simulink model "Section2_b"  (R2023b)
settings: Solver=VariableStepAuto  StartTime=0.0  StopTime=20.0  RelTol=1e-3
settings Model: Creator=paria  LastModifiedBy=paria

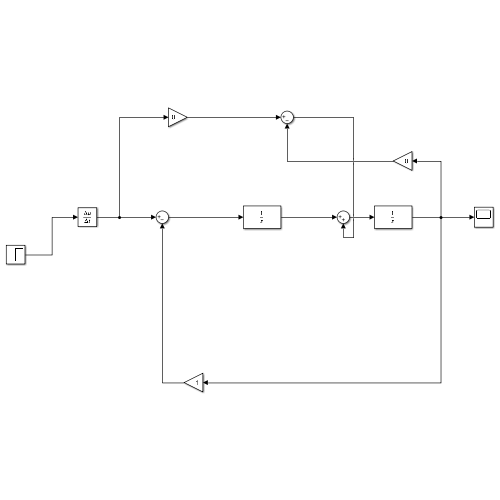
[thumbnail: Simulink's stored preview of the top-level diagram]
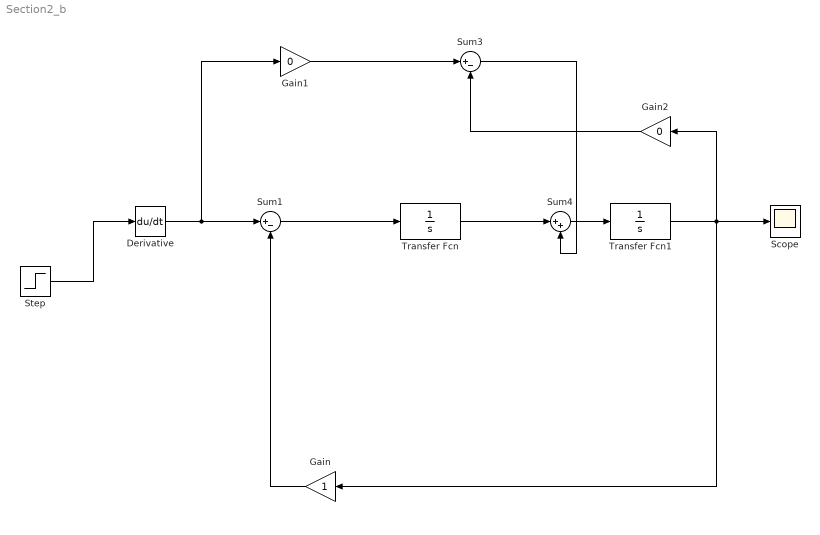
== system Section2_b ==
  Derivative : Derivative
  Gain : Gain
  Gain1 : Gain  Gain=0
  Gain2 : Gain  Gain=0
  Scope : Scope
  Step : Step  Time=0.01  SampleTime=0
  Sum1 : Sum  Inputs=|+-
  Sum3 : Sum  Inputs=|+-
  Sum4 : Sum  Inputs=|++
  Transfer Fcn : TransferFcn  Denominator=[1 0]
  Transfer Fcn1 : TransferFcn  Denominator=[1 0]
  wires:
  Transfer Fcn/1 -> Sum4/1
  Transfer Fcn1/1 -> Gain2/1, Scope/1, Gain/1
  Gain/1 -> Sum1/2
  Gain2/1 -> Sum3/2
  Sum4/1 -> Transfer Fcn1/1
  Step/1 -> Derivative/1
  Sum1/1 -> Transfer Fcn/1
  Sum3/1 -> Sum4/2
  Derivative/1 -> Gain1/1, Sum1/1
  Gain1/1 -> Sum3/1
